simulink model "Velo_BF_PID"  (R2018a)
settings: Solver=VariableStepAuto  StartTime=0.0  StopTime=10.0  RelTol=1e-3
undefined symbols (not defined in the file): Kd_v, Ki_v, Kp_v
libraries: simulink x1
settings Model: Creator=chsira  LastModifiedBy=charl
settings DebuggingCC: LibraryContextMissingDiagnostic=warning
settings SFSimCC: SimUseLocalCustomCode=on
settings RTWCC: RTWUseLocalCustomCode=on

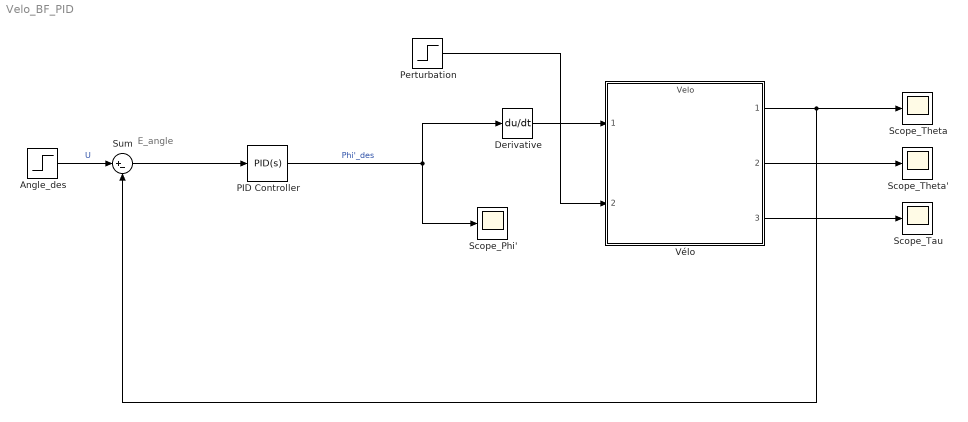
== system Velo_BF_PID ==
  note: E_angle
  "Angle_des " : Step  Time=0  After=0  SampleTime=0
  Derivative : Derivative
  PID Controller : simulink/Continuous/PID Controller  Controller=PID  TimeDomain=Continuous-time  SampleTime=-1  IntegratorMethod=Forward Euler  FilterMethod=Forward Euler  Form=Parallel  UseFilter=on  ControllerParametersSource=internal  P=Kp_v  I=Ki_v  D=Kd_v  N=1  InitialConditionSource=internal  InitialConditionForIntegrator=0  InitialConditionForFilter=0  ExternalReset=none  LimitOutput=off  UpperSaturationLimit=inf  LowerSaturationLimit=-inf  LinearizeAsGain=on  AntiWindupMode=none  Kb=1  TrackingMode=off  Kt=1  PParamMin=[]  PParamMax=[]  IParamMin=[]  IParamMax=[]  DParamMin=[]  DParamMax=[]  NParamMin=[]  NParamMax=[]  KbParamMin=[]  KbParamMax=[]  KtParamMin=[]  KtParamMax=[]  POutMin=[]  POutMax=[]  IOutMin=[]  IOutMax=[]  DOutMin=[]  DOutMax=[]  NOutMin=[]  NOutMax=[]  KbOutMin=[]  KbOutMax=[]  KtOutMin=[]  KtOutMax=[]  IntegratorOutMin=[]  IntegratorOutMax=[]  FilterOutMin=[]  FilterOutMax=[]  SumOutMin=[]  SumOutMax=[]  SumI1OutMin=[]  SumI1OutMax=[]  SumI2OutMin=[]  SumI2OutMax=[]  SumI3OutMin=[]  SumI3OutMax=[]  SumDOutMin=[]  SumDOutMax=[]  SaturationOutMin=[]  SaturationOutMax=[]  IntegratorContinuousStateAttributes=''  IntegratorStateMustResolveToSignalObject=off  IntegratorRTWStateStorageClass=Auto  FilterContinuousStateAttributes=''  FilterStateMustResolveToSignalObject=off  FilterRTWStateStorageClass=Auto  DifferentiatorICPrevScaledInput=0  DifferentiatorOutMin=[]  DifferentiatorOutMax=[]  FilterDiffOutCoefMin=[]  FilterDiffOutCoefMax=[]  SumDenOutMin=[]  SumDenOutMax=[]  SumNumOutMin=[]  SumNumOutMax=[]  ReciprocalOutMin=[]  ReciprocalOutMax=[]  DivideOutMin=[]  DivideOutMax=[]  TunerSelectOption=Transfer Function Based (PID Tuner App)
  Perturbation : Step  Time=0  After=0  SampleTime=0
  "Scope_Phi' " : Scope
  Scope_Tau : Scope
  Scope_Theta : Scope
  Scope_Theta' : Scope
  Sum : Sum  Inputs=|+-
  Vélo : ModelReference  ModelNameDialog=Velo.slx  ParameterArgumentNames=InitialCondition  ParameterArgumentValues=InitialCondition  UsingDefaultArgumentValue=0  SimulationMode=Normal  ModelReferenceVersion=1.22  InitialCondition=5*pi/180  SimulationMode=Normal
  wires:
  Vélo/1 -> Sum/2, Scope_Theta/1
  "Angle_des "/1 -> Sum/1  "U"
  Derivative/1 -> Vélo/1
  Sum/1 -> PID Controller/1
  PID Controller/1 -> Derivative/1, "Scope_Phi' "/1  "Phi'_des"
  Vélo/2 -> Scope_Theta'/1
  Vélo/3 -> Scope_Tau/1
  Perturbation/1 -> Vélo/2
